simulink model "P3_Reconstruccion_de_Seniales"  (R2020a)
settings: Solver=FixedStepDiscrete  StartTime=0.0  StopTime=25  FixedStep=0.001  RelTol=1e-3
undefined symbols (not defined in the file): tripuls
libraries: dsparch4 x2
settings Model: Creator=León Mora  LastModifiedBy=León Mora

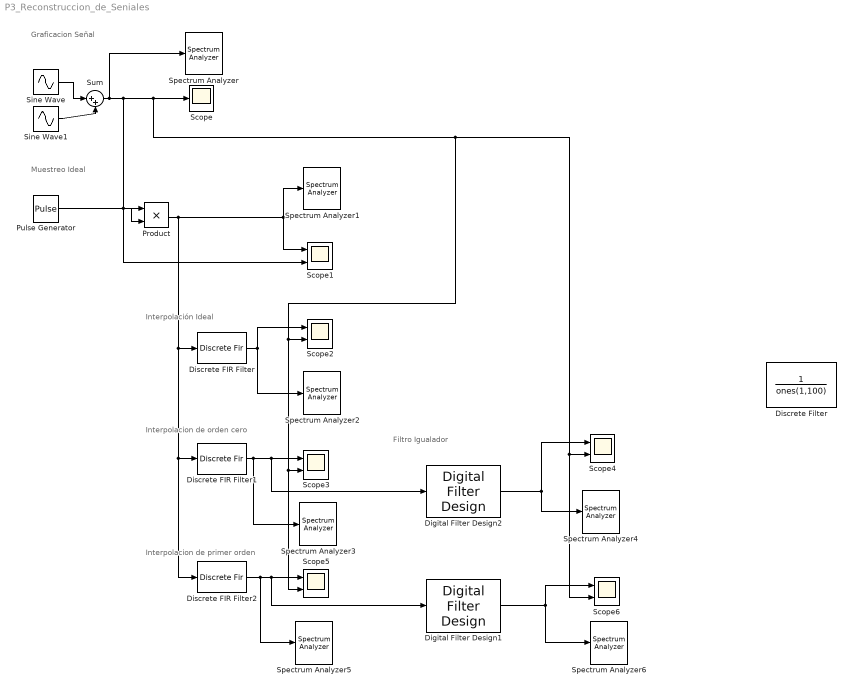
== system P3_Reconstruccion_de_Seniales ==
  note: Filtro Igualador
  note: Interpolacion de primer orden
  note: Interpolacion de orden cero
  note: Interpolación Ideal
  note: Muestreo Ideal
  note: Graficacion Señal
  Digital Filter Design1 : dsparch4/Digital Filter Design  mwdsp_browser_bugfix_var=off
  Digital Filter Design2 : dsparch4/Digital Filter Design  mwdsp_browser_bugfix_var=off
  Discrete FIR Filter : DiscreteFir  Coefficients=sinc([-5:1e-3:5]/0.1)  SampleTime=1e-3
  Discrete FIR Filter1 : DiscreteFir  Coefficients=ones(1,100)  SampleTime=1e-3
  Discrete FIR Filter2 : DiscreteFir  Coefficients=tripuls([-.1:1e-3:.1],0.2)  SampleTime=1e-3
  Discrete Filter : DiscreteFilter  Numerator=1  Denominator=ones(1,100)  InputProcessing=Columns as channels (frame based)  FilterStructure=Direct form II transposed  a0EqualsOne=on
  Product : Product
  Pulse Generator : DiscretePulseGenerator  PulseType=Time based  Period=0.1
  Scope : Scope
  Scope{1..6} (6 alike) : Scope  NumInputPorts=2
  Sine Wave : Sin  Frequency=2*pi  SampleTime=1e-3
  Sine Wave1 : Sin  Frequency=6*pi  SampleTime=1e-3
  Spectrum Analyzer{,1..6} (7 alike) : SpectrumAnalyzer
  Sum : Sum  Inputs=|++
  wires:
  Sine Wave/1 -> Sum/1
  Sine Wave1/1 -> Sum/2
  Sum/1 -> Spectrum Analyzer/1, Product/1, Scope1/2, Scope6/2, Scope4/2, Scope2/2, Scope5/2, Scope3/2, Scope/1
  Pulse Generator/1 -> Product/2
  Product/1 -> Spectrum Analyzer1/1, Scope1/1, Discrete FIR Filter2/1, Discrete FIR Filter1/1, Discrete FIR Filter/1
  Discrete FIR Filter/1 -> Spectrum Analyzer2/1, Scope2/1
  Discrete FIR Filter1/1 -> Digital Filter Design2/1, Scope3/1, Spectrum Analyzer3/1
  Digital Filter Design2/1 -> Spectrum Analyzer4/1, Scope4/1
  Discrete FIR Filter2/1 -> Spectrum Analyzer5/1, Digital Filter Design1/1, Scope5/1
  Digital Filter Design1/1 -> Spectrum Analyzer6/1, Scope6/1
